simulink model "Subsystem2"  (R2023b)
settings: Solver=FixedStepAuto  StartTime=0.0  StopTime=10.0  FixedStep=5e-7  RelTol=1e-3
libraries: mcbcontrolslib x3, dspfdesign x3, slpidlib x3, simulink x1, spsSVPWMGenerator2LevelLib x1
settings Model: Creator=LZQ  LastModifiedBy=LZQ
settings SolverCC: AllowMultiTaskInputOutput=on  ConcurrentTasks=on  AutoInsertRateTranBlk=on
settings DataIOCC: SaveOutput=off  SaveTime=off

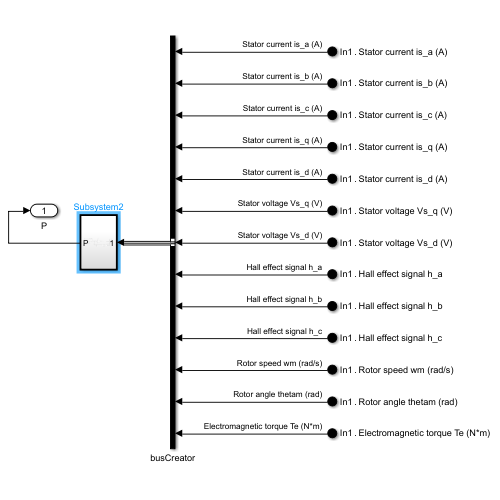
[thumbnail: Simulink's stored preview of the top-level diagram]
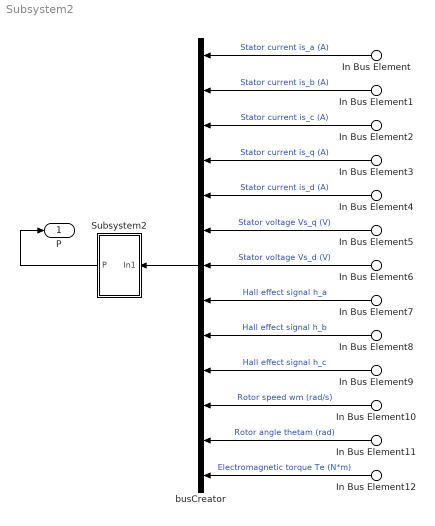
== system Subsystem2 ==
  In Bus Element : Inport  PortName=In1  Element=Stator current is_a (A)
  In Bus Element1 : Inport  PortName=In1  Element=Stator current is_b (A)
  In Bus Element2 : Inport  PortName=In1  Element=Stator current is_c (A)
  In Bus Element3 : Inport  PortName=In1  Element=Stator current is_q (A)
  In Bus Element4 : Inport  PortName=In1  Element=Stator current is_d (A)
  In Bus Element5 : Inport  PortName=In1  Element=Stator voltage Vs_q (V)
  In Bus Element6 : Inport  PortName=In1  Element=Stator voltage Vs_d (V)
  In Bus Element7 : Inport  PortName=In1  Element=Hall effect signal h_a
  In Bus Element8 : Inport  PortName=In1  Element=Hall effect signal h_b
  In Bus Element9 : Inport  PortName=In1  Element=Hall effect signal h_c
  In Bus Element10 : Inport  PortName=In1  Element=Rotor speed wm (rad/s)
  In Bus Element11 : Inport  PortName=In1  Element=Rotor angle thetam (rad)
  In Bus Element12 : Inport  PortName=In1  Element=Electromagnetic torque Te (N*m)
  Subsystem2 : Subsystem  TreatAsAtomicUnit=on
  busCreator : BusCreator  Inputs=13
  P : Outport  OutDataTypeStr=double  PortDimensions=6  SampleTime=0
  wires:
  In Bus Element7/1 -> busCreator/8  "Hall effect signal h_a"
  Subsystem2/1(P) -> P/1
  In Bus Element11/1 -> busCreator/12  "Rotor angle thetam (rad)"
  busCreator/1 -> Subsystem2/1(In1)
  In Bus Element/1 -> busCreator/1  "Stator current is_a (A)"
  In Bus Element1/1 -> busCreator/2  "Stator current is_b (A)"
  In Bus Element3/1 -> busCreator/4  "Stator current is_q (A)"
  In Bus Element2/1 -> busCreator/3  "Stator current is_c (A)"
  In Bus Element4/1 -> busCreator/5  "Stator current is_d (A)"
  In Bus Element5/1 -> busCreator/6  "Stator voltage Vs_q (V)"
  In Bus Element8/1 -> busCreator/9  "Hall effect signal h_b"
  In Bus Element6/1 -> busCreator/7  "Stator voltage Vs_d (V)"
  In Bus Element9/1 -> busCreator/10  "Hall effect signal h_c"
  In Bus Element10/1 -> busCreator/11  "Rotor speed wm (rad/s)"
  In Bus Element12/1 -> busCreator/13  "Electromagnetic torque Te (N*m)"

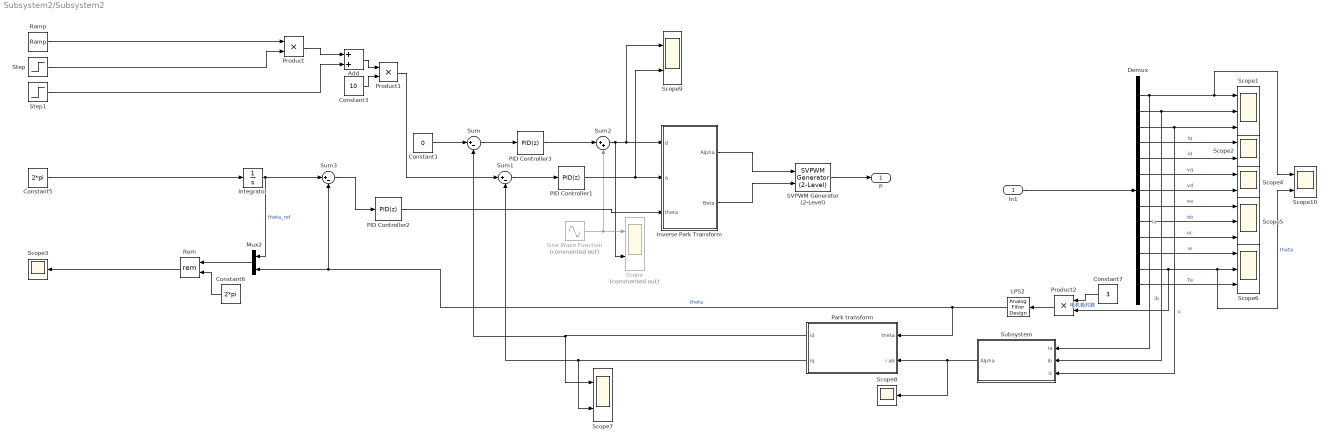
== system Subsystem2/Subsystem2 ==
  In1 : Inport
  Add : Sum
  Constant1 : Constant  Value=0
  Constant3 : Constant  Value=10
  Constant5 : Constant  Value=2*pi
  Constant6 : Constant  Value=2*pi
  Constant7 : Constant  Value=3
  Demux : Demux  Outputs=13
  Integrator : Integrator
  Inverse Park Transform : Subsystem
  LPS2 : dspfdesign/Analog Filter Design  method=Butterworth  filttype=Lowpass  N=8  Wlo=30  Whi=80  Rp=2  Rs=40
  Mux2 : Mux  Inputs=2
  PID Controller1 : slpidlib/PID Controller  Controller=PID  Form=Parallel  TimeDomain=Discrete-time  UseExternalTs=off  SampleTime=1e-5  IntegratorMethod=Forward Euler  FilterMethod=Forward Euler  ControllerParametersSource=internal  P=0.000004  I=0.000001  UseKiTs=off  D=0  N=100  UseFilter=on  TunerSelectOption=Transfer Function Based (PID Tuner App)  InitialConditionSource=internal  InitialConditionForIntegrator=0  InitialConditionForFilter=0  DifferentiatorICPrevScaledInput=0  ExternalReset=none  TrackingMode=off  Kt=1  LimitOutput=off  SatLimitsSource=internal  UpperSaturationLimit=inf  LowerSaturationLimit=-inf  LinearizeAsGain=on  AntiWindupMode=none  Kb=1  LimitIntegrator=off  UpperIntegratorSaturationLimit=inf  LowerIntegratorSaturationLimit=-inf  POutMin=[]  POutMax=[]  IOutMin=[-0.001]  IOutMax=[0.001]  DOutMin=[]  DOutMax=[]  NOutMin=[]  NOutMax=[]  SumOutMin=[-0.01]  SumOutMax=[0.01]  SaturationOutMin=[]  SaturationOutMax=[]  PParamMin=[]  PParamMax=[]  IParamMin=[]  IParamMax=[]  DParamMin=[]  DParamMax=[]  NParamMin=[]  NParamMax=[]  KbParamMin=[]  KbParamMax=[]  KtParamMin=[]  KtParamMax=[]  KbOutMin=[]  KbOutMax=[]  KtOutMin=[]  KtOutMax=[]  IntegratorOutMin=[]  IntegratorOutMax=[]  FilterOutMin=[]  FilterOutMax=[]  SumI1OutMin=[]  SumI1OutMax=[]  SumI2OutMin=[]  SumI2OutMax=[]  SumI3OutMin=[]  SumI3OutMax=[]  SumI4OutMin=[]  SumI4OutMax=[]  SumDOutMin=[]  SumDOutMax=[]  DifferentiatorOutMin=[]  DifferentiatorOutMax=[]  FilterDiffOutCoefMin=[]  FilterDiffOutCoefMax=[]  ReciprocalOutMin=[]  ReciprocalOutMax=[]  SumDenOutMin=[]  SumDenOutMax=[]  SumNumOutMin=[]  SumNumOutMax=[]  DivideOutMin=[]  DivideOutMax=[]  UdiffTsProdOutMin=[]  UdiffTsProdOutMax=[]  NTsProdOutMin=[]  NTsProdOutMax=[]  UintegralTsProdOutMin=[]  UintegralTsProdOutMax=[]  UngainTsProdOutMin=[]  UngainTsProdOutMax=[]  ClampingZeroOutDataTypeStr=Inherit: Inherit via back propagation  ClampingZeroOutMin=[]  ClampingZeroOutMax=[]  FilterDenConstantOutDataTypeStr=Inherit: Inherit via back propagation  FilterDenConstantOutMin=[]  FilterDenConstantOutMax=[]  PCopyOutDataTypeStr=Inherit: Inherit via back propagation  PCopyOutMin=[]  PCopyOutMax=[]  NCopyOutDataTypeStr=Inherit: Inherit via back propagation  NCopyOutMin=[]  NCopyOutMax=[]  IntegratorContinuousStateAttributes=''  IntegratorStateMustResolveToSignalObject=off  IntegratorRTWStateStorageClass=Auto  FilterContinuousStateAttributes=''  FilterStateMustResolveToSignalObject=off  FilterRTWStateStorageClass=Auto  ParallelPVariant=InternalParameters  IdealPVariant=Disabled  IVariant=InternalParameters  DVariant=InternalParameters  IntegratorVariant=Discrete  SatVariant=Disabled  AWVariant=Passthrough  PCopyVariant=Disabled  TRVariant=Disabled  FdbkBlocksVariant=Forward  IdealPFdbkVariant=Disabled  SatFdbkVariant=Disabled  DerivativeFilterVariant=ForwardEulerFilter  NVariant=InternalParameters  NCopyVariant=Disabled  FilterICVariant=InternalICsFilter  IntegratorICVariant=InternalICs  ExternalResetVariant=Disabled  TRSumVariant=Passthrough  SumFdbkVariant=Disabled  SumVariant=Sum_PID  TsampFilterVariant=InternalTs  TsampNgainVariant=Passthrough  TsampIntegralVariant=Disabled_SignalSpec  ExternalSaturationOutDataTypeStr=Inherit: Same as second input
  PID Controller2 : slpidlib/PID Controller  Controller=PID  Form=Parallel  TimeDomain=Discrete-time  UseExternalTs=off  SampleTime=0.0005  IntegratorMethod=Forward Euler  FilterMethod=Forward Euler  ControllerParametersSource=internal  P=0.1  I=0.04  UseKiTs=off  D=0  N=100  UseFilter=on  TunerSelectOption=Transfer Function Based (PID Tuner App)  InitialConditionSource=internal  InitialConditionForIntegrator=0  InitialConditionForFilter=0  DifferentiatorICPrevScaledInput=0  ExternalReset=none  TrackingMode=off  Kt=1  LimitOutput=off  SatLimitsSource=internal  UpperSaturationLimit=inf  LowerSaturationLimit=-inf  LinearizeAsGain=on  AntiWindupMode=none  Kb=1  LimitIntegrator=off  UpperIntegratorSaturationLimit=inf  LowerIntegratorSaturationLimit=-inf  POutMin=[]  POutMax=[]  IOutMin=[]  IOutMax=[]  DOutMin=[]  DOutMax=[]  NOutMin=[]  NOutMax=[]  SumOutMin=[]  SumOutMax=[]  SaturationOutMin=[]  SaturationOutMax=[]  PParamMin=[]  PParamMax=[]  IParamMin=[]  IParamMax=[]  DParamMin=[]  DParamMax=[]  NParamMin=[]  NParamMax=[]  KbParamMin=[]  KbParamMax=[]  KtParamMin=[]  KtParamMax=[]  KbOutMin=[]  KbOutMax=[]  KtOutMin=[]  KtOutMax=[]  IntegratorOutMin=[]  IntegratorOutMax=[]  FilterOutMin=[]  FilterOutMax=[]  SumI1OutMin=[]  SumI1OutMax=[]  SumI2OutMin=[]  SumI2OutMax=[]  SumI3OutMin=[]  SumI3OutMax=[]  SumI4OutMin=[]  SumI4OutMax=[]  SumDOutMin=[]  SumDOutMax=[]  DifferentiatorOutMin=[]  DifferentiatorOutMax=[]  FilterDiffOutCoefMin=[]  FilterDiffOutCoefMax=[]  ReciprocalOutMin=[]  ReciprocalOutMax=[]  SumDenOutMin=[]  SumDenOutMax=[]  SumNumOutMin=[]  SumNumOutMax=[]  DivideOutMin=[]  DivideOutMax=[]  UdiffTsProdOutMin=[]  UdiffTsProdOutMax=[]  NTsProdOutMin=[]  NTsProdOutMax=[]  UintegralTsProdOutMin=[]  UintegralTsProdOutMax=[]  UngainTsProdOutMin=[]  UngainTsProdOutMax=[]  ClampingZeroOutDataTypeStr=Inherit: Inherit via back propagation  ClampingZeroOutMin=[]  ClampingZeroOutMax=[]  FilterDenConstantOutDataTypeStr=Inherit: Inherit via back propagation  FilterDenConstantOutMin=[]  FilterDenConstantOutMax=[]  PCopyOutDataTypeStr=Inherit: Inherit via back propagation  PCopyOutMin=[]  PCopyOutMax=[]  NCopyOutDataTypeStr=Inherit: Inherit via back propagation  NCopyOutMin=[]  NCopyOutMax=[]  IntegratorContinuousStateAttributes=''  IntegratorStateMustResolveToSignalObject=off  IntegratorRTWStateStorageClass=Auto  FilterContinuousStateAttributes=''  FilterStateMustResolveToSignalObject=off  FilterRTWStateStorageClass=Auto  ParallelPVariant=InternalParameters  IdealPVariant=Disabled  IVariant=InternalParameters  DVariant=InternalParameters  IntegratorVariant=Discrete  SatVariant=Disabled  AWVariant=Passthrough  PCopyVariant=Disabled  TRVariant=Disabled  FdbkBlocksVariant=Forward  IdealPFdbkVariant=Disabled  SatFdbkVariant=Disabled  DerivativeFilterVariant=ForwardEulerFilter  NVariant=InternalParameters  NCopyVariant=Disabled  FilterICVariant=InternalICsFilter  IntegratorICVariant=InternalICs  ExternalResetVariant=Disabled  TRSumVariant=Passthrough  SumFdbkVariant=Disabled  SumVariant=Sum_PID  TsampFilterVariant=InternalTs  TsampNgainVariant=Passthrough  TsampIntegralVariant=Disabled_SignalSpec  ExternalSaturationOutDataTypeStr=Inherit: Same as second input
  PID Controller3 : slpidlib/PID Controller  Controller=PID  Form=Parallel  TimeDomain=Discrete-time  UseExternalTs=off  SampleTime=1e-5  IntegratorMethod=Forward Euler  FilterMethod=Forward Euler  ControllerParametersSource=internal  P=0.000004  I=0.000001  UseKiTs=off  D=0  N=100  UseFilter=on  TunerSelectOption=Transfer Function Based (PID Tuner App)  InitialConditionSource=internal  InitialConditionForIntegrator=0  InitialConditionForFilter=0  DifferentiatorICPrevScaledInput=0  ExternalReset=none  TrackingMode=off  Kt=1  LimitOutput=off  SatLimitsSource=internal  UpperSaturationLimit=inf  LowerSaturationLimit=-inf  LinearizeAsGain=on  AntiWindupMode=none  Kb=1  LimitIntegrator=off  UpperIntegratorSaturationLimit=inf  LowerIntegratorSaturationLimit=-inf  POutMin=[]  POutMax=[]  IOutMin=[-0.001]  IOutMax=[0.001]  DOutMin=[]  DOutMax=[]  NOutMin=[]  NOutMax=[]  SumOutMin=[-0.01]  SumOutMax=[0.01]  SaturationOutMin=[]  SaturationOutMax=[]  PParamMin=[]  PParamMax=[]  IParamMin=[]  IParamMax=[]  DParamMin=[]  DParamMax=[]  NParamMin=[]  NParamMax=[]  KbParamMin=[]  KbParamMax=[]  KtParamMin=[]  KtParamMax=[]  KbOutMin=[]  KbOutMax=[]  KtOutMin=[]  KtOutMax=[]  IntegratorOutMin=[]  IntegratorOutMax=[]  FilterOutMin=[]  FilterOutMax=[]  SumI1OutMin=[]  SumI1OutMax=[]  SumI2OutMin=[]  SumI2OutMax=[]  SumI3OutMin=[]  SumI3OutMax=[]  SumI4OutMin=[]  SumI4OutMax=[]  SumDOutMin=[]  SumDOutMax=[]  DifferentiatorOutMin=[]  DifferentiatorOutMax=[]  FilterDiffOutCoefMin=[]  FilterDiffOutCoefMax=[]  ReciprocalOutMin=[]  ReciprocalOutMax=[]  SumDenOutMin=[]  SumDenOutMax=[]  SumNumOutMin=[]  SumNumOutMax=[]  DivideOutMin=[]  DivideOutMax=[]  UdiffTsProdOutMin=[]  UdiffTsProdOutMax=[]  NTsProdOutMin=[]  NTsProdOutMax=[]  UintegralTsProdOutMin=[]  UintegralTsProdOutMax=[]  UngainTsProdOutMin=[]  UngainTsProdOutMax=[]  ClampingZeroOutDataTypeStr=Inherit: Inherit via back propagation  ClampingZeroOutMin=[]  ClampingZeroOutMax=[]  FilterDenConstantOutDataTypeStr=Inherit: Inherit via back propagation  FilterDenConstantOutMin=[]  FilterDenConstantOutMax=[]  PCopyOutDataTypeStr=Inherit: Inherit via back propagation  PCopyOutMin=[]  PCopyOutMax=[]  NCopyOutDataTypeStr=Inherit: Inherit via back propagation  NCopyOutMin=[]  NCopyOutMax=[]  IntegratorContinuousStateAttributes=''  IntegratorStateMustResolveToSignalObject=off  IntegratorRTWStateStorageClass=Auto  FilterContinuousStateAttributes=''  FilterStateMustResolveToSignalObject=off  FilterRTWStateStorageClass=Auto  ParallelPVariant=InternalParameters  IdealPVariant=Disabled  IVariant=InternalParameters  DVariant=InternalParameters  IntegratorVariant=Discrete  SatVariant=Disabled  AWVariant=Passthrough  PCopyVariant=Disabled  TRVariant=Disabled  FdbkBlocksVariant=Forward  IdealPFdbkVariant=Disabled  SatFdbkVariant=Disabled  DerivativeFilterVariant=ForwardEulerFilter  NVariant=InternalParameters  NCopyVariant=Disabled  FilterICVariant=InternalICsFilter  IntegratorICVariant=InternalICs  ExternalResetVariant=Disabled  TRSumVariant=Passthrough  SumFdbkVariant=Disabled  SumVariant=Sum_PID  TsampFilterVariant=InternalTs  TsampNgainVariant=Passthrough  TsampIntegralVariant=Disabled_SignalSpec  ExternalSaturationOutDataTypeStr=Inherit: Same as second input
  Park transform : Subsystem
  Product : Product
  Product1 : Product
  Product2 : Product
  Ramp : simulink/Sources/Ramp  slope=0.2  start=0  InitialOutput=0.2
  Rem : Math  Operator=rem
  SVPWM Generator (2-Level) : spsSVPWMGenerator2LevelLib/SVPWM Generator (2-Level)  InputType=alpha-beta components  SwitchingPattern=Pattern #1  Fc=20000  ParUref=[0.8 -30 50]  Ts=0
  Scope : Scope  Commented=on  NumInputPorts=2
  Scope1 : Scope  NumInputPorts=3
  Scope{2,4,7,9..10} (5 alike) : Scope  NumInputPorts=2
  Scope3 : Scope
  Scope5 : Scope  NumInputPorts=3
  Scope6 : Scope  NumInputPorts=3
  Scope8 : Scope
  Sine Wave Function : Sin  Commented=on  Amplitude=0.2  Frequency=2*pi*800  Phase=pi/2  SampleTime=0.000005
  Step : Step  Time=4  Before=1  After=0  SampleTime=0
  Step1 : Step  Time=4  SampleTime=0
  Subsystem : Subsystem
  Sum : Sum  Inputs=|+-
  Sum1 : Sum  Inputs=|+-
  Sum2 : Sum  Inputs=|++
  Sum3 : Sum  Inputs=|+-
  P : Outport
  wires:
  In1/1 -> Demux/1
  SVPWM Generator (2-Level)/1 -> P/1
  Product2/1 -> LPS2/1
  Step/1 -> Product/2
  Sum/1 -> PID Controller3/1
  Product1/1 -> Sum1/1
  Demux/8 -> Scope5/1  "ea"
  Demux/5 -> Scope2/2  "id"
  Demux/6 -> Scope4/1  "vq"
  Demux/11 -> Scope6/1  "w"
  Constant6/1 -> Rem/2
  Mux2/1 -> Rem/1
  Demux/10 -> Scope5/3  "ec"
  Ramp/1 -> Product/1
  Subsystem/1(Alpha) -> Scope8/1, Park transform/2(i ab)
  Demux/13 -> Scope6/3  "Te"
  Step1/1 -> Add/2
  Demux/2 -> Scope1/2, Subsystem/2(ib)  "ib"
  Demux/4 -> Scope2/1  "iq"
  Integrator/1 -> Sum3/1, Mux2/1  "theta_ref"
  Demux/3 -> Scope1/3, Subsystem/3(ic)  "ic"
  Add/1 -> Product1/1
  Constant5/1 -> Integrator/1
  Demux/12 -> Scope6/2, Scope10/2, Product2/2  "theta"
  Park transform/1(id) -> Scope7/1, Sum/2
  Constant7/1 -> Product2/1  "电机极对数"
  Sum3/1 -> PID Controller2/1
  Sum1/1 -> PID Controller1/1
  Park transform/2(iq) -> Scope7/2, Sum1/2
  PID Controller3/1 -> Sum2/1
  Product/1 -> Add/1
  Constant1/1 -> Sum/1
  Inverse Park Transform/2(Beta) -> SVPWM Generator (2-Level)/2
  Demux/7 -> Scope4/2  "vd"
  Sum2/1 -> Scope/2, Inverse Park Transform/1(d), Scope9/1
  Constant3/1 -> Product1/2
  Rem/1 -> Scope3/1
  Demux/9 -> Scope5/2  "eb"
  Sine Wave Function/1 -> Scope/1, Sum2/2
  Inverse Park Transform/1(Alpha) -> SVPWM Generator (2-Level)/1
  LPS2/1 -> Park transform/1(theta), Mux2/2, Sum3/2  "theta"
  PID Controller1/1 -> Inverse Park Transform/2(q), Scope9/2
  Demux/1 -> Scope1/1, Scope10/1, Subsystem/1(ia)  "ia"
  PID Controller2/1 -> Inverse Park Transform/3(theta)

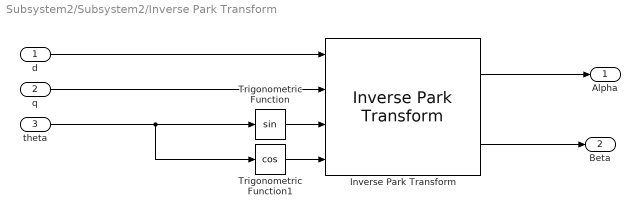
== system Subsystem2/Subsystem2/Inverse Park Transform ==
  d : Inport
  q : Inport  Port=2
  theta : Inport  Port=3
  Inverse Park Transform : mcbcontrolslib/Inverse Park Transform  PhaseInput=Two inputs  AxisAlignment=D-axis  ThetaInput=Sine and Cosine electrical position  AngleInput=Per-unit  N_points=1024
      settings: LibrarySourceBlock=mcblib/Controls/Math Transforms/Inverse Park Transform
  Trigonometric Function : Trigonometry
  Trigonometric Function1 : Trigonometry  Operator=cos
  Alpha : Outport
  Beta : Outport  Port=2
  wires:
  Inverse Park Transform/2 -> Beta/1
  q/1 -> Inverse Park Transform/2
  d/1 -> Inverse Park Transform/1
  Inverse Park Transform/1 -> Alpha/1
  Trigonometric Function/1 -> Inverse Park Transform/3
  Trigonometric Function1/1 -> Inverse Park Transform/4
  theta/1 -> Trigonometric Function/1, Trigonometric Function1/1

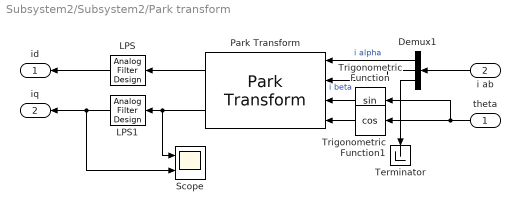
== system Subsystem2/Subsystem2/Park transform ==
  theta : Inport  SampleTime=1e-5
  i ab : Inport  Port=2  SampleTime=1e-5
  Demux1 : Demux  Outputs=3
  LPS : dspfdesign/Analog Filter Design  method=Butterworth  filttype=Lowpass  N=3  Wlo=500  Whi=80  Rp=2  Rs=40
  LPS1 : dspfdesign/Analog Filter Design  method=Butterworth  filttype=Lowpass  N=3  Wlo=500  Whi=80  Rp=2  Rs=40
  Park Transform : mcbcontrolslib/Park Transform  PhaseInput=Two inputs  AxisAlignment=D-axis  ThetaInput=Sine and Cosine electrical position  AngleInput=Per-unit  N_points=1024
      settings: LibrarySourceBlock=mcblib/Controls/Math Transforms/Park Transform
  Scope : Scope  NumInputPorts=2
  Terminator : Terminator
  Trigonometric Function : Trigonometry
  Trigonometric Function1 : Trigonometry  Operator=cos
  id : Outport  SampleTime=1e-5
  iq : Outport  Port=2  SampleTime=1e-5
  wires:
  LPS1/1 -> Scope/2, iq/1
  i ab/1 -> Demux1/1
  Trigonometric Function/1 -> Park Transform/3
  Demux1/1 -> Park Transform/1  "i alpha"
  Demux1/2 -> Park Transform/2  "i beta"
  Park Transform/2 -> LPS1/1, Scope/1
  LPS/1 -> id/1
  Park Transform/1 -> LPS/1
  theta/1 -> Trigonometric Function1/1, Trigonometric Function/1
  Trigonometric Function1/1 -> Park Transform/4
  Demux1/3 -> Terminator/1

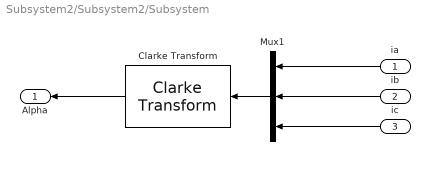
== system Subsystem2/Subsystem2/Subsystem ==
  ia : Inport  SampleTime=1e-5
  ib : Inport  Port=2  SampleTime=1e-5
  ic : Inport  Port=3  SampleTime=1e-5
  Clarke Transform : mcbcontrolslib/Clarke Transform  VariantControl=Variant2  PhaseInput=Three inputs  EnPowerInv=off
      settings: LibrarySourceBlock=mcblib/Controls/Math Transforms/Clarke Transform
  Mux1 : Mux  Inputs=3
  Alpha : Outport  SampleTime=1e-5
  wires:
  ic/1 -> Mux1/3
  Clarke Transform/1 -> Alpha/1
  ib/1 -> Mux1/2
  ia/1 -> Mux1/1
  Mux1/1 -> Clarke Transform/1
